simulink model "untitled"  (R2016b)
settings: Solver=ode4  StartTime=0.0  StopTime=inf  FixedStep=0.002  RelTol=1e-3  EnableMultiTasking=on
settings Model: SimulationMode=external  Creator=zczg  LastModifiedBy=zczg
settings SolverCC: EnableConcurrentExecution=on
settings DataIOCC: SaveFormat=StructureWithTime
settings OptimizationCC: BlockReduction=off  OptimizeBlockIOStorage=off  BufferReuse=off  GlobalBufferReuse=off  ExpressionFolding=off  LocalBlockOutputs=off
settings HardwareCC: ProdBitPerPointer=32  ProdBitPerSizeT=32  ProdBitPerPtrDiffT=32  ProdLargestAtomicFloat=None  ProdWordSize=32  ProdLongLongMode=on  ProdHWDeviceType=Generic->32-bit x86 compatible
settings RTWCC: SystemTargetFile=slrt.tlc  TemplateMakefile=slrt_default_tmf  Description=Simulink Real-Time  RTWCompilerOptimization=on

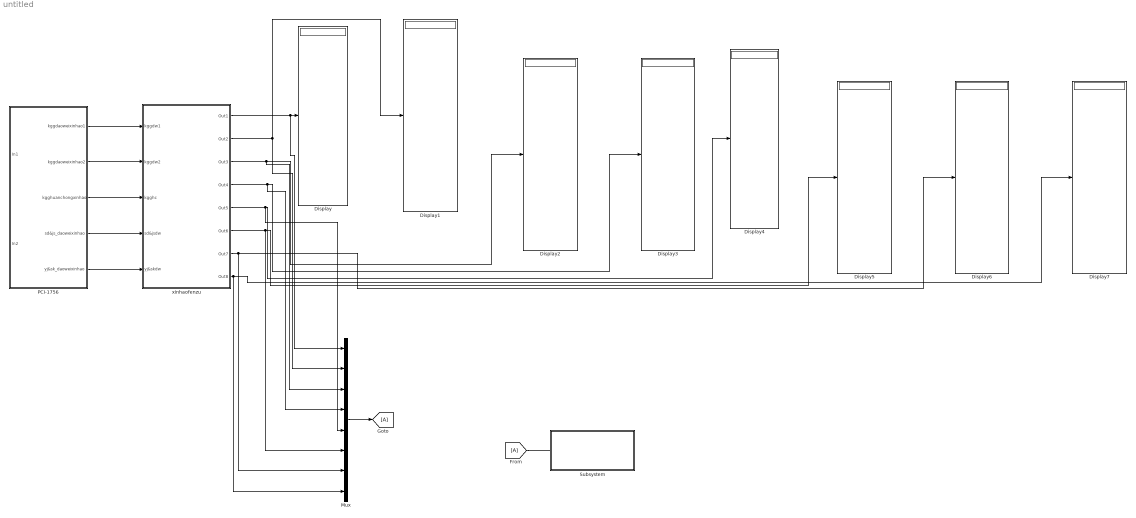
== system untitled ==
  Display{,1..7} (8 alike) : Display
  Mux : Mux  Inputs=8
  PCI-1756 : Subsystem
  Subsystem : Subsystem
  xinhaofenzu : Subsystem
  wires:
  PCI-1756/1(kggdaoweixinhao1) -> xinhaofenzu/1(kggdw1)
  PCI-1756/2(kggdaoweixinhao2) -> xinhaofenzu/2(kggdw2)
  PCI-1756/3(kgghuanchongxinhao) -> xinhaofenzu/3(kgghc)
  PCI-1756/4(sd&js_daoweixinhao) -> xinhaofenzu/4(sd&jsdw)
  PCI-1756/5(yj&sk_daoweixinhao) -> xinhaofenzu/5(yj&skdw)
  xinhaofenzu/1(Out1) -> Mux/1, Display/1
  xinhaofenzu/2(Out2) -> Mux/2, Display1/1
  xinhaofenzu/3(Out3) -> Mux/3, Display2/1
  xinhaofenzu/4(Out4) -> Mux/4, Display3/1
  xinhaofenzu/5(Out5) -> Mux/5, Display4/1
  xinhaofenzu/6(Out6) -> Mux/6, Display5/1
  xinhaofenzu/7(Out7) -> Mux/7, Display6/1
  xinhaofenzu/8(Out8) -> Mux/8, Display7/1
  Mux/1 -> [A]
  [A] -> ?

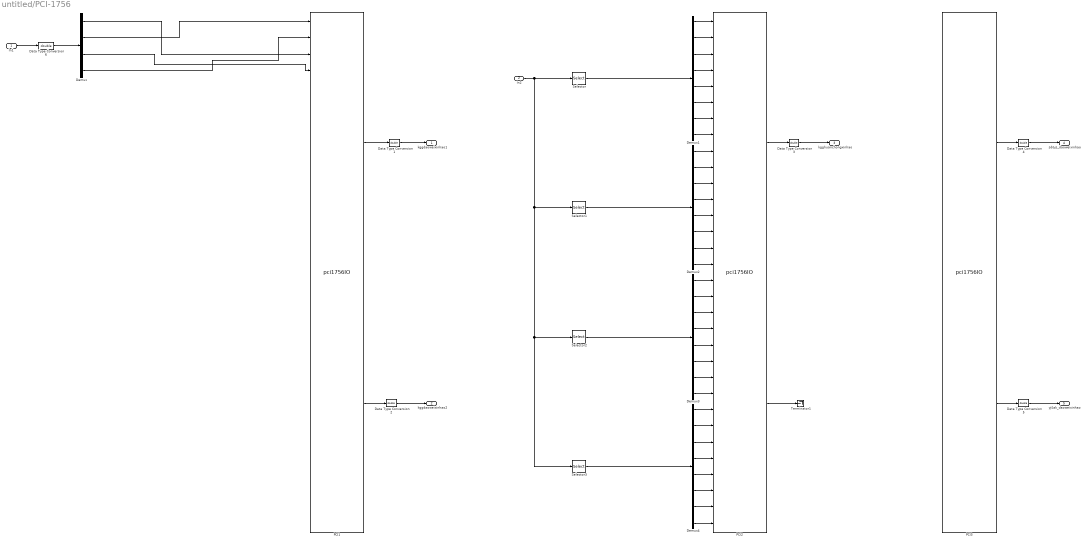
== system untitled/PCI-1756 ==
  In1 : Inport
  In2 : Inport  Port=2
  Data Type Conversion{1..6} (6 alike) : DataTypeConversion  OutDataTypeStr=double
  Demux : Demux
  Demux{1..4} (4 alike) : Demux  Outputs=8
  PCI1 : S-Function  FunctionName=pci1756IO  Parameters=[SampleTime SampleOffset], SLOT  SFunctionDeploymentMode=off  EnableBusSupport=off  mask(PCI1756){Sample=0.002, SLOT=[4 13]}
      mask prompts: Sample "Sample time:"
      mask help:
      | PCI-1756
      | Advantech
      | Digital Input&Output
      mask init:
      | SampleTime =0.002; SampleOffset=0;
      mask Display:
      | disp('PCI1756\nDigital output&input\n');
      | port_label('input',1,'DO1');
      | port_label('input',2,'DO2');
      | port_label('input',3,'DO3');
      | port_label('input',4,'DO4');
      | port_label('input',5,'DO5');
      | port_label('input',6,'DO6');
      | port_label('input',7,'DO7');
      | port_label('input',8,'DO8');
      | port_label('input',9,'DO9');
      | port_label('input',10,'DO10');
      | port_label('input',11,'DO11');
      | port_label('input',12,'DO12');
      | port_label('input',13,'DO13');
      | port_label('input',14,'DO14');
      | port_label('input',15,'DO15');
      | port_label('input',16,'DO16');
      | port_label('input',17,'DO17');
      | port_label('input',18,'DO18');
      | port_label('input',19,'DO19');
      | port_label('input',20,'DO20');
      | port_label('input',21,'DO21');
      | port_label('input',22,'DO22');
      | port_label('input',23,'DO23');
      | port_label('input',24,'DO24');
      | port_label('input',25,'DO25');
      | port_label('input',26,'DO26');
      | port_label('input',27,'DO27');
      | port_label('input',28,'DO28');
      | port_label('input',29,'DO29');
      | port_label('input',30,'DO30');
      | port_label('input',31,'DO31');
      | port_label('input',32,'DO32');
      | port_label('output',1,'DI1');
      | port_label('output',2,'DI2');
  PCI2 : S-Function  FunctionName=pci1756IO  Parameters=[SampleTime SampleOffset], SLOT  SFunctionDeploymentMode=off  EnableBusSupport=off  mask(PCI1756){Sample=0.002, SLOT=[4 14]}
      mask prompts: Sample "Sample time:"
      mask help:
      | PCI-1756
      | Advantech
      | Digital Input&Output
      mask init:
      | SampleTime =0.002; SampleOffset=0;
      mask Display:
      | disp('PCI1756\nDigital output&input\n');
      | port_label('input',1,'DO1');
      | port_label('input',2,'DO2');
      | port_label('input',3,'DO3');
      | port_label('input',4,'DO4');
      | port_label('input',5,'DO5');
      | port_label('input',6,'DO6');
      | port_label('input',7,'DO7');
      | port_label('input',8,'DO8');
      | port_label('input',9,'DO9');
      | port_label('input',10,'DO10');
      | port_label('input',11,'DO11');
      | port_label('input',12,'DO12');
      | port_label('input',13,'DO13');
      | port_label('input',14,'DO14');
      | port_label('input',15,'DO15');
      | port_label('input',16,'DO16');
      | port_label('input',17,'DO17');
      | port_label('input',18,'DO18');
      | port_label('input',19,'DO19');
      | port_label('input',20,'DO20');
      | port_label('input',21,'DO21');
      | port_label('input',22,'DO22');
      | port_label('input',23,'DO23');
      | port_label('input',24,'DO24');
      | port_label('input',25,'DO25');
      | port_label('input',26,'DO26');
      | port_label('input',27,'DO27');
      | port_label('input',28,'DO28');
      | port_label('input',29,'DO29');
      | port_label('input',30,'DO30');
      | port_label('input',31,'DO31');
      | port_label('input',32,'DO32');
      | port_label('output',1,'DI1');
      | port_label('output',2,'DI2');
  PCI3 : S-Function  FunctionName=pci1756IO  Parameters=[SampleTime SampleOffset], SLOT  SFunctionDeploymentMode=off  EnableBusSupport=off  mask(PCI1756){Sample=0.002, SLOT=[4 15]}
      mask prompts: Sample "Sample time:"
      mask help:
      | PCI-1756
      | Advantech
      | Digital Input&Output
      mask init:
      | SampleTime =0.002; SampleOffset=0;
      mask Display:
      | disp('PCI1756\nDigital output&input\n');
      | port_label('input',1,'DO1');
      | port_label('input',2,'DO2');
      | port_label('input',3,'DO3');
      | port_label('input',4,'DO4');
      | port_label('input',5,'DO5');
      | port_label('input',6,'DO6');
      | port_label('input',7,'DO7');
      | port_label('input',8,'DO8');
      | port_label('input',9,'DO9');
      | port_label('input',10,'DO10');
      | port_label('input',11,'DO11');
      | port_label('input',12,'DO12');
      | port_label('input',13,'DO13');
      | port_label('input',14,'DO14');
      | port_label('input',15,'DO15');
      | port_label('input',16,'DO16');
      | port_label('input',17,'DO17');
      | port_label('input',18,'DO18');
      | port_label('input',19,'DO19');
      | port_label('input',20,'DO20');
      | port_label('input',21,'DO21');
      | port_label('input',22,'DO22');
      | port_label('input',23,'DO23');
      | port_label('input',24,'DO24');
      | port_label('input',25,'DO25');
      | port_label('input',26,'DO26');
      | port_label('input',27,'DO27');
      | port_label('input',28,'DO28');
      | port_label('input',29,'DO29');
      | port_label('input',30,'DO30');
      | port_label('input',31,'DO31');
      | port_label('input',32,'DO32');
      | port_label('output',1,'DI1');
      | port_label('output',2,'DI2');
  Selector : Selector  InputPortWidth=32  IndexOptions=Index vector (dialog)  Indices=[1 5 9 13 17 21 25 29]  OutputSizes=1
  Selector1 : Selector  InputPortWidth=32  IndexOptions=Index vector (dialog)  Indices=[2 6 10 14 18 22 26 30]  OutputSizes=1
  Selector2 : Selector  InputPortWidth=32  IndexOptions=Index vector (dialog)  Indices=[3 7 11 15 19 23 27 31]  OutputSizes=1
  Selector3 : Selector  InputPortWidth=32  IndexOptions=Index vector (dialog)  Indices=[4 8 12 16 20 24 28 32]  OutputSizes=1
  Terminator1 : Terminator
  kggdaoweixinhao1 : Outport
  kggdaoweixinhao2 : Outport  Port=2
  kgghuanchongxinhao : Outport  Port=3
  sd&js_daoweixinhao : Outport  Port=4
  yj&sk_daoweixinhao : Outport  Port=5
  wires:
  PCI1/1 -> Data Type Conversion1/1
  Data Type Conversion1/1 -> kggdaoweixinhao1/1
  PCI1/2 -> Data Type Conversion2/1
  Data Type Conversion2/1 -> kggdaoweixinhao2/1
  PCI2/2 -> Terminator1/1
  PCI2/1 -> Data Type Conversion3/1
  Data Type Conversion3/1 -> kgghuanchongxinhao/1
  PCI3/1 -> Data Type Conversion4/1
  Data Type Conversion4/1 -> sd&js_daoweixinhao/1
  Data Type Conversion5/1 -> yj&sk_daoweixinhao/1
  PCI3/2 -> Data Type Conversion5/1
  In1/1 -> Data Type Conversion6/1
  Demux1/8 -> PCI2/8
  Demux1/7 -> PCI2/7
  Demux1/6 -> PCI2/6
  Demux1/5 -> PCI2/5
  Demux1/4 -> PCI2/4
  Demux1/3 -> PCI2/3
  Demux1/2 -> PCI2/2
  Demux1/1 -> PCI2/1
  Selector/1 -> Demux1/1
  Demux2/8 -> PCI2/16
  Demux2/7 -> PCI2/15
  Demux2/6 -> PCI2/14
  Demux2/5 -> PCI2/13
  Demux2/4 -> PCI2/12
  Demux2/3 -> PCI2/11
  Demux2/2 -> PCI2/10
  Demux2/1 -> PCI2/9
  Demux3/8 -> PCI2/24
  Demux3/7 -> PCI2/23
  Demux3/6 -> PCI2/22
  Demux3/5 -> PCI2/21
  Demux3/4 -> PCI2/20
  Demux3/3 -> PCI2/19
  Demux3/2 -> PCI2/18
  Demux3/1 -> PCI2/17
  Demux4/8 -> PCI2/32
  Demux4/7 -> PCI2/31
  Demux4/6 -> PCI2/30
  Demux4/5 -> PCI2/29
  Demux4/4 -> PCI2/28
  Demux4/3 -> PCI2/27
  Demux4/2 -> PCI2/26
  Demux4/1 -> PCI2/25
  Selector1/1 -> Demux2/1
  Selector2/1 -> Demux3/1
  Selector3/1 -> Demux4/1
  In2/1 -> Selector3/1, Selector2/1, Selector1/1, Selector/1
  Demux/1 -> PCI1/3
  Demux/2 -> PCI1/1
  Demux/3 -> PCI1/4
  Demux/4 -> PCI1/2
  Data Type Conversion6/1 -> Demux/1

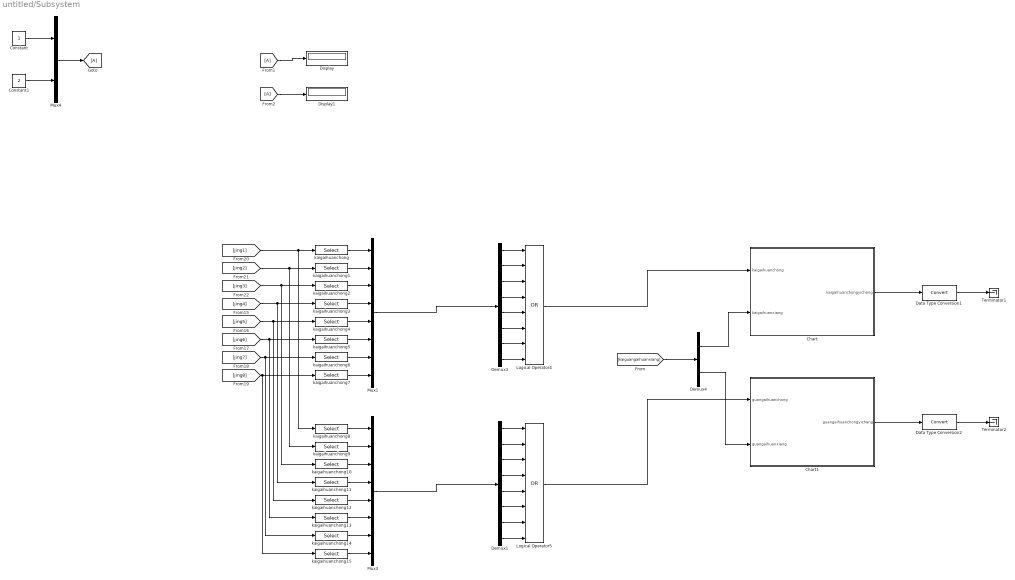
== system untitled/Subsystem ==
  Chart : Stateflow chart  TreatAsAtomicUnit=on
  Chart1 : Stateflow chart  TreatAsAtomicUnit=on
  Constant : Constant
  Constant1 : Constant  Value=2
  Data Type Conversion1 : DataTypeConversion
  Data Type Conversion2 : DataTypeConversion
  Demux1 : Demux  Outputs=8
  Demux3 : Demux  Outputs=8
  Demux4 : Demux  Outputs=2
  Display : Display
  Display1 : Display
  Logical Operator4 : Logic  Operator=OR  Inputs=8  AllPortsSameDT=off  OutDataTypeStr=boolean
  Logical Operator5 : Logic  Operator=OR  Inputs=8  AllPortsSameDT=off  OutDataTypeStr=boolean
  Mux1 : Mux  Inputs=8
  Mux3 : Mux  Inputs=8
  Mux4 : Mux  Inputs=2
  Terminator1 : Terminator
  Terminator2 : Terminator
  kaigaihuanchong{,1..7} (8 alike) : Selector  IndexOptions=Index vector (dialog)  Indices=[5]  OutputSizes=1
  kaigaihuanchong{8..15} (8 alike) : Selector  IndexOptions=Index vector (dialog)  Indices=[6]  OutputSizes=1
  wires:
  Constant1/1 -> Mux4/2
  Constant/1 -> Mux4/1
  Mux4/1 -> [A]
  [A] -> Display/1
  [A] -> Display1/1
  Demux3/1 -> Logical Operator4/1
  Demux3/3 -> Logical Operator4/3
  Demux3/4 -> Logical Operator4/4
  Demux3/5 -> Logical Operator4/5
  Demux3/2 -> Logical Operator4/2
  Demux3/6 -> Logical Operator4/6
  Demux3/7 -> Logical Operator4/7
  Demux3/8 -> Logical Operator4/8
  Demux1/1 -> Logical Operator5/1
  Demux1/3 -> Logical Operator5/3
  Demux1/4 -> Logical Operator5/4
  Demux1/5 -> Logical Operator5/5
  Demux1/2 -> Logical Operator5/2
  Demux1/6 -> Logical Operator5/6
  Demux1/7 -> Logical Operator5/7
  Demux1/8 -> Logical Operator5/8
  Logical Operator4/1 -> Chart/1(kaigaihuanchong)
  [kaiguangaihuanxiang] -> Demux4/1
  Demux4/1 -> Chart/2(kaigaihuanxiang)
  Logical Operator5/1 -> Chart1/1(guangaihuanchong)
  Demux4/2 -> Chart1/2(guangaihuanxiang)
  Chart1/1(guangaihuanchongyichang) -> Data Type Conversion2/1
  Chart/1(kaigaihuanchongyichang) -> Data Type Conversion1/1
  Data Type Conversion1/1 -> Terminator1/1
  Data Type Conversion2/1 -> Terminator2/1
  kaigaihuanchong/1 -> Mux1/1
  kaigaihuanchong1/1 -> Mux1/2
  kaigaihuanchong2/1 -> Mux1/3
  kaigaihuanchong3/1 -> Mux1/4
  kaigaihuanchong4/1 -> Mux1/5
  kaigaihuanchong5/1 -> Mux1/6
  kaigaihuanchong6/1 -> Mux1/7
  kaigaihuanchong7/1 -> Mux1/8
  Mux1/1 -> Demux3/1
  [jing1] -> kaigaihuanchong8/1, kaigaihuanchong/1
  [jing2] -> kaigaihuanchong9/1, kaigaihuanchong1/1
  [jing3] -> kaigaihuanchong10/1, kaigaihuanchong2/1
  [jing4] -> kaigaihuanchong11/1, kaigaihuanchong3/1
  [jing5] -> kaigaihuanchong12/1, kaigaihuanchong4/1
  [jing6] -> kaigaihuanchong13/1, kaigaihuanchong5/1
  [jing7] -> kaigaihuanchong14/1, kaigaihuanchong6/1
  [jing8] -> kaigaihuanchong15/1, kaigaihuanchong7/1
  kaigaihuanchong8/1 -> Mux3/1
  kaigaihuanchong9/1 -> Mux3/2
  kaigaihuanchong10/1 -> Mux3/3
  kaigaihuanchong11/1 -> Mux3/4
  kaigaihuanchong12/1 -> Mux3/5
  kaigaihuanchong13/1 -> Mux3/6
  kaigaihuanchong14/1 -> Mux3/7
  kaigaihuanchong15/1 -> Mux3/8
  Mux3/1 -> Demux1/1

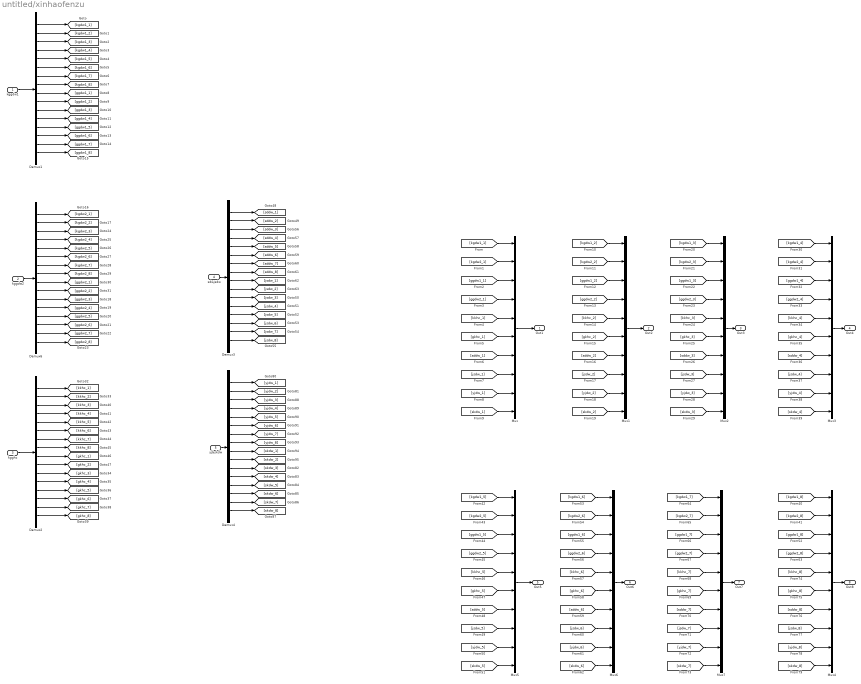
== system untitled/xinhaofenzu ==
  kggdw1 : Inport
  kggdw2 : Inport  Port=2
  kgghc : Inport  Port=3
  sd&jsdw : Inport  Port=4
  yj&skdw : Inport  Port=5
  Demux{1..4,6} (5 alike) : Demux  Outputs=16
  Mux{,1..7} (8 alike) : Mux  Inputs=10
  Out1 : Outport
  Out2 : Outport  Port=2
  Out3 : Outport  Port=3
  Out4 : Outport  Port=4
  Out5 : Outport  Port=5
  Out6 : Outport  Port=6
  Out7 : Outport  Port=7
  Out8 : Outport  Port=8
  wires:
  kggdw1/1 -> Demux1/1
  sd&jsdw/1 -> Demux3/1
  Mux/1 -> Out1/1
  Mux1/1 -> Out2/1
  kggdw2/1 -> Demux6/1
  kgghc/1 -> Demux2/1
  yj&skdw/1 -> Demux4/1
  Demux1/1 -> [kgdw1_1]
  Demux1/2 -> [kgdw1_2]
  Demux1/3 -> [kgdw1_3]
  Demux1/4 -> [kgdw1_4]
  Demux1/5 -> [kgdw1_5]
  Demux1/6 -> [kgdw1_6]
  Demux1/7 -> [kgdw1_7]
  Demux1/8 -> [kgdw1_8]
  Demux1/9 -> [ggdw1_1]
  Demux1/10 -> [ggdw1_2]
  Demux1/11 -> [ggdw1_3]
  Demux1/12 -> [ggdw1_4]
  Demux1/13 -> [ggdw1_5]
  Demux1/14 -> [ggdw1_6]
  Demux1/15 -> [ggdw1_7]
  Demux1/16 -> [ggdw1_8]
  Demux6/1 -> [kgdw2_1]
  Demux6/2 -> [kgdw2_2]
  Demux6/3 -> [kgdw2_3]
  Demux6/4 -> [kgdw2_4]
  Demux6/5 -> [kgdw2_5]
  Demux6/6 -> [kgdw2_6]
  Demux6/7 -> [kgdw2_7]
  Demux6/8 -> [kgdw2_8]
  Demux6/9 -> [ggdw2_1]
  Demux6/10 -> [ggdw2_2]
  Demux6/11 -> [ggdw2_3]
  Demux6/12 -> [ggdw2_4]
  Demux6/13 -> [ggdw2_5]
  Demux6/14 -> [ggdw2_6]
  Demux6/15 -> [ggdw2_7]
  Demux6/16 -> [ggdw2_8]
  Demux2/1 -> [kkhc_1]
  Demux2/2 -> [kkhc_2]
  Demux2/3 -> [kkhc_3]
  Demux2/4 -> [kkhc_4]
  Demux2/5 -> [kkhc_5]
  Demux2/6 -> [kkhc_6]
  Demux2/7 -> [kkhc_7]
  Demux2/8 -> [kkhc_8]
  Demux2/9 -> [gkhc_1]
  Demux2/10 -> [gkhc_2]
  Demux2/11 -> [gkhc_3]
  Demux2/12 -> [gkhc_4]
  Demux2/13 -> [gkhc_5]
  Demux2/14 -> [gkhc_6]
  Demux2/15 -> [gkhc_7]
  Demux2/16 -> [gkhc_8]
  Demux3/1 -> [sddw_1]
  Demux3/2 -> [sddw_2]
  Demux3/3 -> [sddw_3]
  Demux3/4 -> [sddw_4]
  Demux3/5 -> [sddw_5]
  Demux3/6 -> [sddw_6]
  Demux3/7 -> [sddw_7]
  Demux3/8 -> [sddw_8]
  Demux3/9 -> [jsdw_1]
  Demux3/16 -> [jsdw_8]
  Demux3/15 -> [jsdw_7]
  Demux3/14 -> [jsdw_6]
  Demux3/13 -> [jsdw_5]
  Demux3/12 -> [jsdw_4]
  Demux3/11 -> [jsdw_3]
  Demux3/10 -> [jsdw_2]
  Demux4/1 -> [yjdw_1]
  Demux4/2 -> [yjdw_2]
  Demux4/3 -> [yjdw_3]
  Demux4/4 -> [yjdw_4]
  Demux4/5 -> [yjdw_5]
  Demux4/6 -> [yjdw_6]
  Demux4/7 -> [yjdw_7]
  Demux4/8 -> [yjdw_8]
  Demux4/9 -> [skdw_1]
  Demux4/16 -> [skdw_8]
  Demux4/15 -> [skdw_7]
  Demux4/14 -> [skdw_6]
  Demux4/13 -> [skdw_5]
  Demux4/12 -> [skdw_4]
  Demux4/11 -> [skdw_3]
  Demux4/10 -> [skdw_2]
  [kgdw1_1] -> Mux/1
  [kgdw2_1] -> Mux/2
  [ggdw1_1] -> Mux/3
  [ggdw2_1] -> Mux/4
  [kkhc_1] -> Mux/5
  [gkhc_1] -> Mux/6
  [sddw_1] -> Mux/7
  [jsdw_1] -> Mux/8
  [yjdw_1] -> Mux/9
  [skdw_1] -> Mux/10
  [kgdw1_2] -> Mux1/1
  [kgdw2_2] -> Mux1/2
  [ggdw1_2] -> Mux1/3
  [ggdw2_2] -> Mux1/4
  [kkhc_2] -> Mux1/5
  [gkhc_2] -> Mux1/6
  [sddw_2] -> Mux1/7
  [jsdw_2] -> Mux1/8
  [yjdw_2] -> Mux1/9
  [skdw_2] -> Mux1/10
  [kgdw1_3] -> Mux2/1
  [kgdw2_3] -> Mux2/2
  [ggdw1_3] -> Mux2/3
  [ggdw2_3] -> Mux2/4
  [kkhc_3] -> Mux2/5
  [gkhc_3] -> Mux2/6
  [sddw_3] -> Mux2/7
  [jsdw_3] -> Mux2/8
  [yjdw_3] -> Mux2/9
  [skdw_3] -> Mux2/10
  [kgdw1_4] -> Mux3/1
  [kgdw2_4] -> Mux3/2
  [ggdw1_4] -> Mux3/3
  [ggdw2_4] -> Mux3/4
  [kkhc_4] -> Mux3/5
  [gkhc_4] -> Mux3/6
  [sddw_4] -> Mux3/7
  [jsdw_4] -> Mux3/8
  [yjdw_4] -> Mux3/9
  [skdw_4] -> Mux3/10
  Mux2/1 -> Out3/1
  Mux3/1 -> Out4/1
  Mux5/1 -> Out5/1
  [kgdw1_5] -> Mux5/1
  [kgdw2_5] -> Mux5/2
  [ggdw1_5] -> Mux5/3
  [ggdw2_5] -> Mux5/4
  [kkhc_5] -> Mux5/5
  [gkhc_5] -> Mux5/6
  [sddw_5] -> Mux5/7
  [jsdw_5] -> Mux5/8
  [yjdw_5] -> Mux5/9
  [skdw_5] -> Mux5/10
  [kgdw1_6] -> Mux6/1
  [kgdw2_6] -> Mux6/2
  [ggdw1_6] -> Mux6/3
  [ggdw2_6] -> Mux6/4
  [kkhc_6] -> Mux6/5
  [gkhc_6] -> Mux6/6
  [sddw_6] -> Mux6/7
  [jsdw_6] -> Mux6/8
  [yjdw_6] -> Mux6/9
  [skdw_6] -> Mux6/10
  [kgdw1_7] -> Mux7/1
  [kgdw2_7] -> Mux7/2
  [ggdw1_7] -> Mux7/3
  [ggdw2_7] -> Mux7/4
  [kkhc_7] -> Mux7/5
  [gkhc_7] -> Mux7/6
  [sddw_7] -> Mux7/7
  [jsdw_7] -> Mux7/8
  [yjdw_7] -> Mux7/9
  [skdw_7] -> Mux7/10
  Mux6/1 -> Out6/1
  Mux7/1 -> Out7/1
  [kgdw1_8] -> Mux4/1
  [kgdw2_8] -> Mux4/2
  [ggdw1_8] -> Mux4/3
  [ggdw2_8] -> Mux4/4
  [kkhc_8] -> Mux4/5
  [gkhc_8] -> Mux4/6
  [sddw_8] -> Mux4/7
  [jsdw_8] -> Mux4/8
  [yjdw_8] -> Mux4/9
  [skdw_8] -> Mux4/10
  Mux4/1 -> Out8/1

== stateflow chart untitled/Subsystem/Chart ==
  state off
    entry:
    kaigaihuanchongyichang=0;
    t=0;
  state on
    entry:
    t=t+0.002;
  state on1
    entry:
    kaigaihuanchongyichang=1;
  (default) -> off
  off -> on : [kaigaihuanxiang==1]
  on -> on [order 1] : [t<=8&&kaigaihuanchong==0]
  on -> on1 [order 2] : [t>8&&kaigaihuanchong==1]
  data: t local; kaigaihuanchongyichang output; kaigaihuanchong input; kaigaihuanxiang input

== stateflow chart untitled/Subsystem/Chart1 ==
  state off
    entry:
    guangaihuanchongyichang=0;
    t=0;
  state on
    entry:
    t=t+0.002;
  state on1
    entry:
    guangaihuanchongyichang=1;
  (default) -> off
  off -> on : [guangaihuanxiang==1]
  on -> on [order 1] : [t<=8&&guangaihuanchong==0]
  on -> on1 [order 2] : [t>8&&guangaihuanchong==1]
  data: guangaihuanchong input; t local; guangaihuanxiang input; guangaihuanchongyichang output
